simulink model "Cart_pendulum_Simulitation"  (R2023b)
settings: Solver=VariableStepAuto  StartTime=0.0  StopTime=10.0  RelTol=1e-3
settings Model: Creator=frede  LastModifiedBy=frede

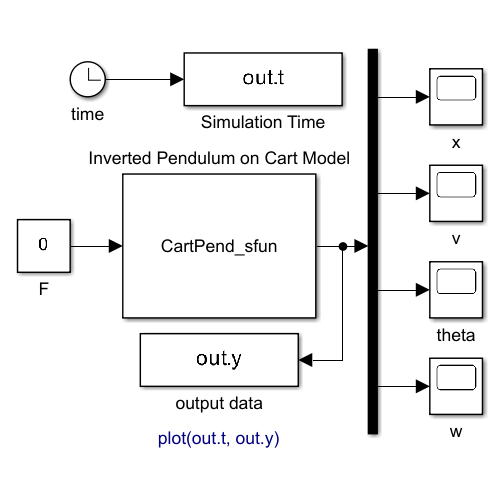
[thumbnail: Simulink's stored preview of the top-level diagram]
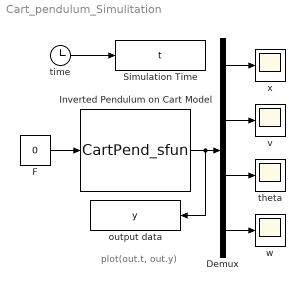
== system Cart_pendulum_Simulitation ==
  note: plot(out.t, out.y)
  Demux : Demux
  F : Constant  Value=0
  Inverted Pendulum on Cart Model : M-S-Function  FunctionName=CartPend_sfun  Parameters=0, 0, pi, .3
  Simulation Time : ToWorkspace  VariableName=t  SampleTime=-1
  output data : ToWorkspace  VariableName=y  SampleTime=-1
  theta : Scope
  time : Clock
  v : Scope
  w : Scope
  x : Scope
  wires:
  F/1 -> Inverted Pendulum on Cart Model/1
  Inverted Pendulum on Cart Model/1 -> output data/1, Demux/1
  Demux/4 -> w/1
  Demux/3 -> theta/1
  Demux/2 -> v/1
  Demux/1 -> x/1
  time/1 -> Simulation Time/1
